simulink model "feedback_harness"  (R2016a)
settings: Solver=ode45  StartTime=0.0  StopTime=4  FixedStep=T_sample_control  RelTol=1e-3
settings Model: ModifiedByFormat=The MathWorks Inc.  Creator=The MathWorks, Inc.  LastModifiedBy=The MathWorks Inc.
settings SolverCC: AlgebraicLoopSolver=LineSearch
settings DataIOCC: LimitDataPoints=on  SaveFormat=Array  SaveOutput=off  SaveTime=off
settings OptimizationCC: ExpressionDepthLimit=2147483647  LifeSpan=1
settings DebuggingCC: UnderspecifiedInitializationDetection=Classic  MergeDetectMultiDrivingBlocksExec=none  SolverPrmCheckMsg=warning  FcnCallInpInsideContextMsg=EnableAllAsWarning  StateNameClashWarn=warning
settings HardwareCC: ProdBitPerPointer=32  ProdLargestAtomicFloat=None  ProdIntDivRoundTo=Undefined  ProdEndianess=Unspecified  ProdWordSize=32  ProdHWDeviceType=32-bit Generic
settings ModelReferenceCC: ModelReferenceMinAlgLoopOccurrences=on  PropagateSignalLabelsOutOfModel=off
settings GRTTargetCC: CombineOutputUpdateFcns=off  GRTInterface=on
settings ConfigComp: CovModelRefEnable=Off  CovSFcnEnable=off

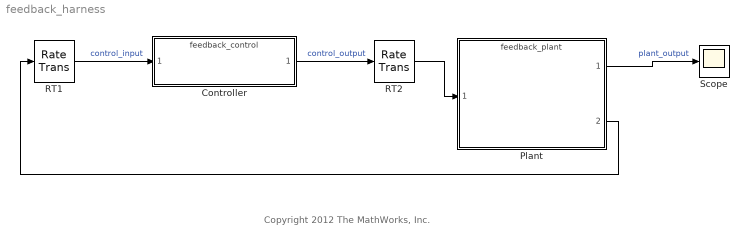
== system feedback_harness ==
  note: Copyright 2012 The MathWorks, Inc.
  Controller : ModelReference  ModelNameDialog=feedback_control.slx  SimulationMode=Normal  ModelReferenceVersion=1.43
  Plant : ModelReference  ModelNameDialog=feedback_plant  SimulationMode=Normal  ModelReferenceVersion=1.28
  RT1 : RateTransition
  RT2 : RateTransition
  Scope : Scope
  wires:
  Plant/2 -> RT1/1
  Controller/1 -> RT2/1  "control_output"
  Plant/1 -> Scope/1  "plant_output"
  RT1/1 -> Controller/1  "control_input"
  RT2/1 -> Plant/1
